simulink model "throttle_body"  (Simulink 3.00)
settings: Solver=ode45  SolverMode=SingleTasking  StartTime=0.0  StopTime=6.5  FixedStep=.0005  RelTol=1e-3  AbsTol=1e-6
settings Model: OutputSaveName=vel  LastModifiedBy=paul

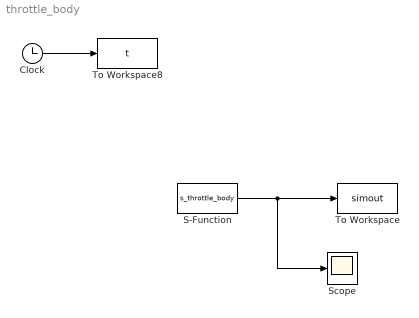
== system throttle_body ==
  Clock : Clock
      settings: DisplayTime=off  Decimation=10
  S-Function : S-Function  FunctionName=s_throttle_body  PortCounts=[]  SFunctionModules=''
  Scope : Scope
      settings: TimeRange=auto  YMin=-5  YMax=5  SaveToWorkspace=off  SaveName=ScopeData
  To Workspace : ToWorkspace  VariableName=simout  SampleTime=-1  SaveFormat=Matrix
  To Workspace8 : ToWorkspace  VariableName=t  SampleTime=-1  SaveFormat=Matrix
  wires:
  Clock/1 -> To Workspace8/1
  S-Function/1 -> To Workspace/1, Scope/1
